simulink model "antenna_ADRC_sim_sol"  (R2023b)
settings: Solver=ode3  StartTime=0.0  StopTime=20  FixedStep=0.01  RelTol=1e-3
values from neighbouring files (symbols this model uses):
  A = [ 0 1 ; 0 -a_m ]    [antenna_ADRC_par_sol.m]    (also in antenna_OFB_par_sol.m; pendulum_ADRC_par_sol.m = [ 0 , 1 , 0 ; 0 , 0 , 1 ; 0 , 0 , 0 ])
  A_ESO = [ 0 , 1 , 0 ; 0 , 0 , 1 ; 0 , 0 , 0 ]    [antenna_ADRC_par_sol.m]
  b = Kl*Kg    (= 10)    [antenna_ADRC_par_sol.m]
  B = [ 0 ; Kl*Kg ]    [antenna_ADRC_par_sol.m]    (also in antenna_OFB_par_sol.m; pendulum_ADRC_par_sol.m = [ 0; b0 ; 0 ])
  B_ESO = [ 0; b ; 0 ]    [antenna_ADRC_par_sol.m]
  C = [ 1 , 0 ]    [antenna_ADRC_par_sol.m]    (also in antenna_OFB_par_sol.m; pendulum_ADRC_par_sol.m = [ 1 , 0 , 0 ])
  C_ESO = [ 1 , 0 , 0 ]    [antenna_ADRC_par_sol.m]
  k1 = K(1)    [antenna_ADRC_par_sol.m]
  k2 = K(2)    [antenna_ADRC_par_sol.m]
  L_ESO = acker(A_ESO',C_ESO',p_ESO)'    [antenna_ADRC_par_sol.m]
libraries: simulink_extras x3
settings Model: Creator=jerome  LastModifiedBy=jerome
settings ModelReferenceCC: EnableRefExpFcnMdlSchedulingChecks=on

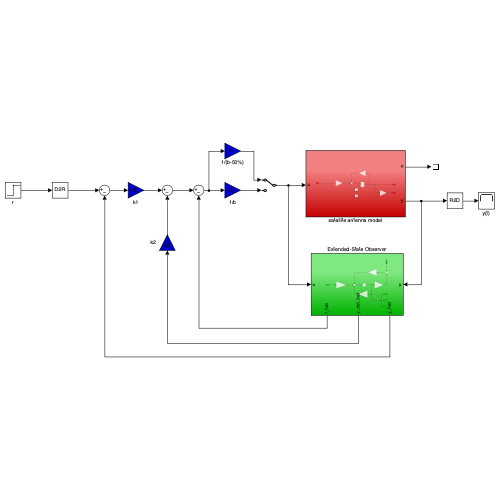
[thumbnail: Simulink's stored preview of the top-level diagram]
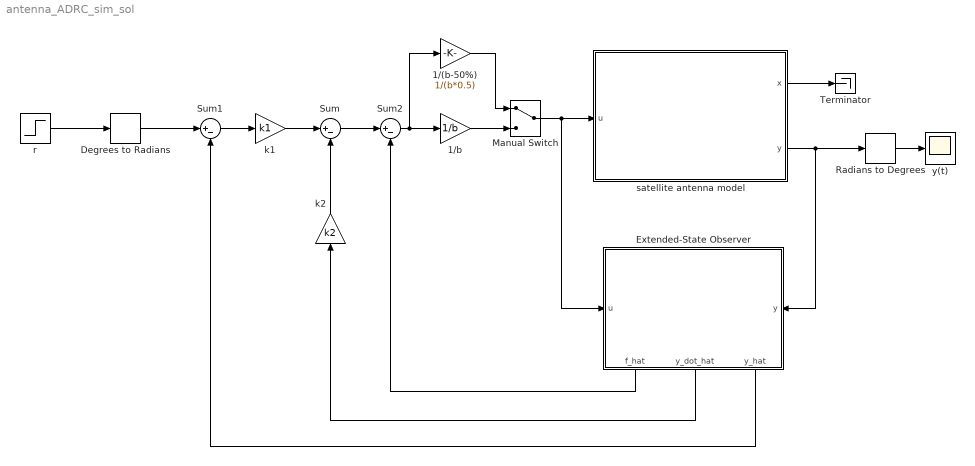
== system antenna_ADRC_sim_sol ==
  1/(b-50%) : Gain  Gain=1/(b*0.5)
  1/b : Gain  Gain=1/b
  Degrees to Radians : simulink_extras/Transformations/Degrees to Radians
  Extended-State Observer : Subsystem
      settings: PortSchema="{\"entries\":[{\"content\":{\"sides\":[{\"content\":{\"connectorIds\":[\"In1\"]},\"type\":\"ConnectorPlacement.EquallySpacedRectSide\",\"uuid\":\"e39c489f-7ce3-4515-bfb3-5978cf16689b\"},{\"content\":{\"connectorIds\":[\"In2\"],\"side\":\"RIGHT\"},\"type\":\"ConnectorPlacement.EquallySpacedRectSide\",\"uuid\":\"c323375b-3042-4327-9d10-0e78d49b9c28\"},{\"content\":{\"connectorIds\":[],\"side\":\"TOP\"},\"type\":\"ConnectorPlacement.EquallySpacedRectSide\",\"uuid\":\"bc6e3c93-589b-408b-8e2a-2332a4933e23\"},{\"content\":{\"connectorIds\":[\"Out1\",\"Out2\",\"Out3\"],\"side\":\"BOTTOM\"},\"type\":\"ConnectorPlacement.EquallySpacedRectSide\",\"uuid\":\"0fa3e6d2-737b-4634-8e4c-4849dc2892cb\"}]},\"type\":\"ConnectorPlacement.EquallySpacedConnector\",\"uuid\":\"052b3b38-b01c-47b0-92b2-1f2c82c768d4\"}],\"packageUris\":[\"http://schema.mathworks.com/mf0/Connector/R2020b\"],\"version\":\"1.0\"}"
  Manual Switch : ManualSwitch
  Radians to Degrees : simulink_extras/Transformations/Radians to Degrees
  Sum : Sum  Inputs=|+-
  Sum1 : Sum  Inputs=|+-
  Sum2 : Sum  Inputs=|+-
  Terminator : Terminator
  k1 : Gain  Gain=k1
  k2 : Gain  Gain=k2
  r : Step  Time=5  Before=30  After=90  SampleTime=0
  satellite antenna model : Subsystem
  y(t) : Scope
  wires:
  Sum2/1 -> 1/(b-50%)/1, 1/b/1
  Extended-State Observer/3(y_hat) -> Sum1/2
  Extended-State Observer/1(f_hat) -> Sum2/2
  k1/1 -> Sum/1
  k2/1 -> Sum/2
  Sum/1 -> Sum2/1
  Sum1/1 -> k1/1
  Extended-State Observer/2(y_dot_hat) -> k2/1
  Degrees to Radians/1 -> Sum1/1
  r/1 -> Degrees to Radians/1
  satellite antenna model/2(y) -> Extended-State Observer/2(y), Radians to Degrees/1
  satellite antenna model/1(x) -> Terminator/1
  Radians to Degrees/1 -> y(t)/1
  1/b/1 -> Manual Switch/2
  Manual Switch/1 -> Extended-State Observer/1(u), satellite antenna model/1(u)
  1/(b-50%)/1 -> Manual Switch/1

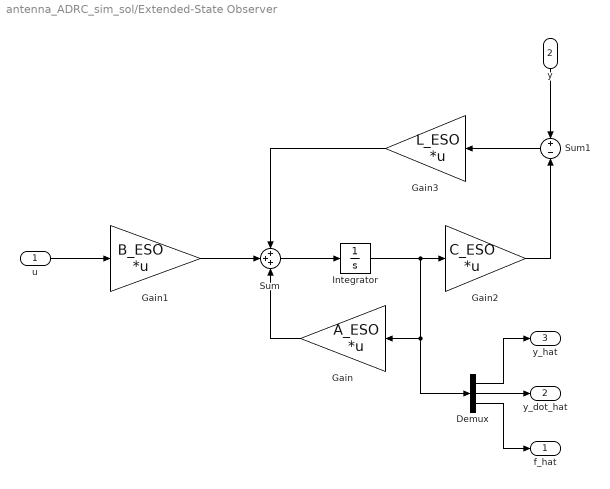
== system antenna_ADRC_sim_sol/Extended-State Observer ==
  u : Inport
  y : Inport  Port=2
  Demux : Demux  Outputs=3
  Gain : Gain  Gain=A_ESO  Multiplication=Matrix(K*u) (u vector)
  Gain1 : Gain  Gain=B_ESO  Multiplication=Matrix(K*u) (u vector)
  Gain2 : Gain  Gain=C_ESO  Multiplication=Matrix(K*u) (u vector)
  Gain3 : Gain  Gain=L_ESO  Multiplication=Matrix(K*u) (u vector)
  Integrator : Integrator  InitialCondition=zeros(3,1)
  Sum : Sum  Inputs=+++
  Sum1 : Sum  Inputs=+-
  f_hat : Outport
  y_dot_hat : Outport  Port=2
  y_hat : Outport  Port=3
  wires:
  Integrator/1 -> Gain2/1, Demux/1, Gain/1
  Demux/1 -> y_hat/1
  Sum/1 -> Integrator/1
  u/1 -> Gain1/1
  Gain/1 -> Sum/3
  Gain1/1 -> Sum/2
  Gain3/1 -> Sum/1
  Sum1/1 -> Gain3/1
  Gain2/1 -> Sum1/2
  y/1 -> Sum1/1
  Demux/3 -> f_hat/1
  Demux/2 -> y_dot_hat/1

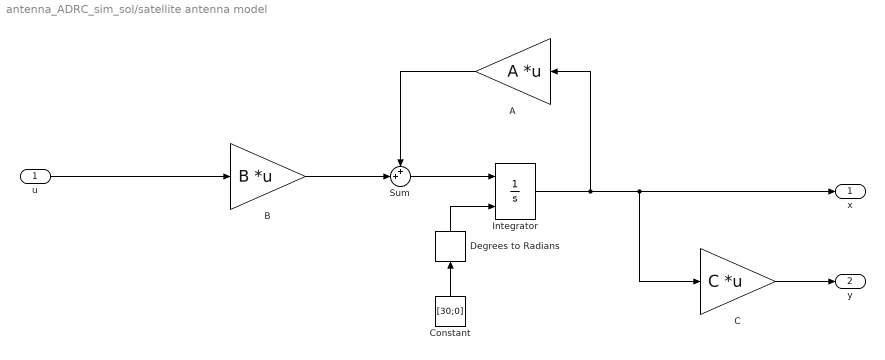
== system antenna_ADRC_sim_sol/satellite antenna model ==
  u : Inport
  A : Gain  Gain=A  Multiplication=Matrix(K*u) (u vector)
  B : Gain  Gain=B  Multiplication=Matrix(K*u) (u vector)
  C : Gain  Gain=C  Multiplication=Matrix(K*u) (u vector)
  Constant : Constant  Value=[30;0]  VectorParams1D=off
  Degrees to Radians : simulink_extras/Transformations/Degrees to Radians
  Integrator : Integrator  InitialConditionSource=external  InitialCondition=[0.1;0]
  Sum : Sum  Inputs=++|
  x : Outport
  y : Outport  Port=2
  wires:
  Sum/1 -> Integrator/1
  Integrator/1 -> A/1, C/1, x/1
  C/1 -> y/1
  Constant/1 -> Degrees to Radians/1
  Degrees to Radians/1 -> Integrator/2
  A/1 -> Sum/1
  B/1 -> Sum/2
  u/1 -> B/1
